simulink model "inverted_pendulum"  (R2019b)
settings: Solver=VariableStepAuto  StartTime=0.0  StopTime=10.0  RelTol=1e-3
settings Model: Creator=mahdie  LastModifiedBy=mahdie

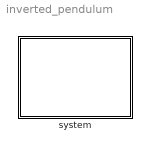
== system inverted_pendulum ==
  system : Subsystem

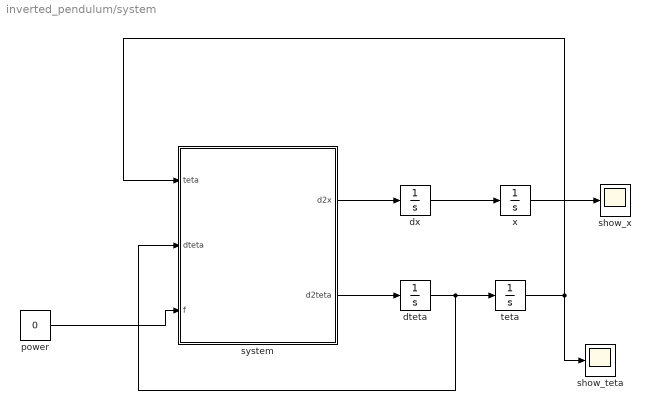
== system inverted_pendulum/system ==
  "dteta " : Integrator
  dx : Integrator
  power : Constant  Value=0
  show_teta : Scope
  show_x : Scope
  "system " : MATLAB Function  TreatAsAtomicUnit=on
  teta : Integrator  InitialCondition=0.1
  x : Integrator
  wires:
  dx/1 -> x/1
  "system "/2(d2teta) -> "dteta "/1
  "system "/1(d2x) -> dx/1
  "dteta "/1 -> "system "/2(dteta), teta/1
  teta/1 -> "system "/1(teta), show_teta/1
  power/1 -> "system "/3(f)
  x/1 -> show_x/1

== matlab function inverted_pendulum/system/system  ==
  data: d2x output; teta input; dteta input; f input; d2teta output
function [d2x,d2teta] = fcn(teta,dteta,f)

k = 1/(l*(M+m)-m*l*cos(teta)^2);
d2teta = (-g*sin(teta)*(M+m)-cos(teta)*(f+m*l*dteta^2*sin(teta)))/k;
d2x = (m*l*g*cos(teta)*sin(teta)+l*(f+m*l*dteta^2*sin(teta)))/k;
